simulink model "Quadrotor_Model"  (R2024b)
settings: Solver=ode45  StartTime=0.0  StopTime=350  RelTol=1e-3  EnableMultiTasking=on
values from neighbouring files (symbols this model uses):
  b = 0.07    [project_launch.m]
  g = 9.81    [project_launch.m]
  Ixx = 0.03411283500000001    (= 0.034112835)    [project_launch.m]
  Iyy = Ixx    (= 0.034112835)    [project_launch.m]
  Izz = 0.06314503500000002    (= 0.063145035)    [project_launch.m]
  Jr = 1.6129e-05    [project_launch.m]
  k = 0.09    [project_launch.m]
  K_d_phi = 0.01    [project_launch.m]
  K_d_psi = 0.136    [project_launch.m]
  K_d_theta = 0.1    [project_launch.m]
  K_dx = 0.00001    (= 1e-05)    [project_launch.m]
  K_dy = 0.00005    (= 5e-05)    [project_launch.m]
  K_dz = 0.001    [project_launch.m]
  K_p_phi = 0.05    [project_launch.m]
  K_p_psi = 0.4    [project_launch.m]
  K_p_theta = 0.0002    [project_launch.m]
  K_px = 0.00003    (= 3e-05)    [project_launch.m]
  K_py = 0.0001    [project_launch.m]
  K_pz = 0.0001    [project_launch.m]
  L = 0.381    [project_launch.m]
  m = 1.8    [project_launch.m]
settings Model: Creator=boyan  LastModifiedBy=Akhil Jarodia
settings SolverCC: MaxConsecutiveMinStep=2  AlgebraicLoopSolver=TrustRegion
settings DataIOCC: LimitDataPoints=on  SaveFormat=Array  ReturnWorkspaceOutputs=off
settings OptimizationCC: LifeSpan=inf
settings DebuggingCC: SolverPrmCheckMsg=warning  UnconnectedInputMsg=warning  UnconnectedOutputMsg=warning  UnconnectedLineMsg=warning  SFUnexpectedBacktrackingDiag=warning  SFNoUnconditionalDefaultTransitionDiag=warning  SFExecutionAtInitializationDiag=none  ArithmeticOperatorsInVariantConditions=warning
settings HardwareCC: ProdBitPerPointer=32  ProdBitPerSizeT=32  ProdBitPerPtrDiffT=32  ProdLargestAtomicFloat=None  ProdIntDivRoundTo=Undefined  ProdEndianess=Unspecified  ProdWordSize=32  ProdHWDeviceType=32-bit Generic
settings ModelReferenceCC: EnableRefExpFcnMdlSchedulingChecks=on  PropagateSignalLabelsOutOfModel=off
settings SFSimCC: SimUseLocalCustomCode=off  CustomCodeUndefinedFunction=UseInterfaceOnly
settings RTWCC: RTWUseLocalCustomCode=off  GPUComputeCapability=3.5  DLArmComputeVersion=19.05
settings CodeAppCC: StateflowObjectComments=on
settings GRTTargetCC: TargetLangStandard=C89/C90 (ANSI)
settings ConfigComp: CovMetricSettings=dw  CovSaveCumulativeToWorkspaceVar=on  CovSaveSingleToWorkspaceVar=on  CovExternalEMLEnable=off  CovSFcnEnable=off

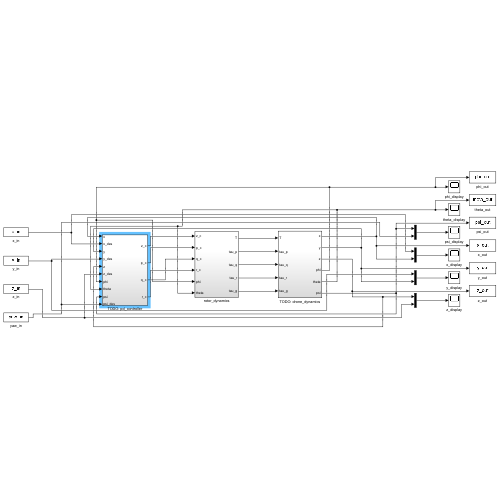
[thumbnail: Simulink's stored preview of the top-level diagram]
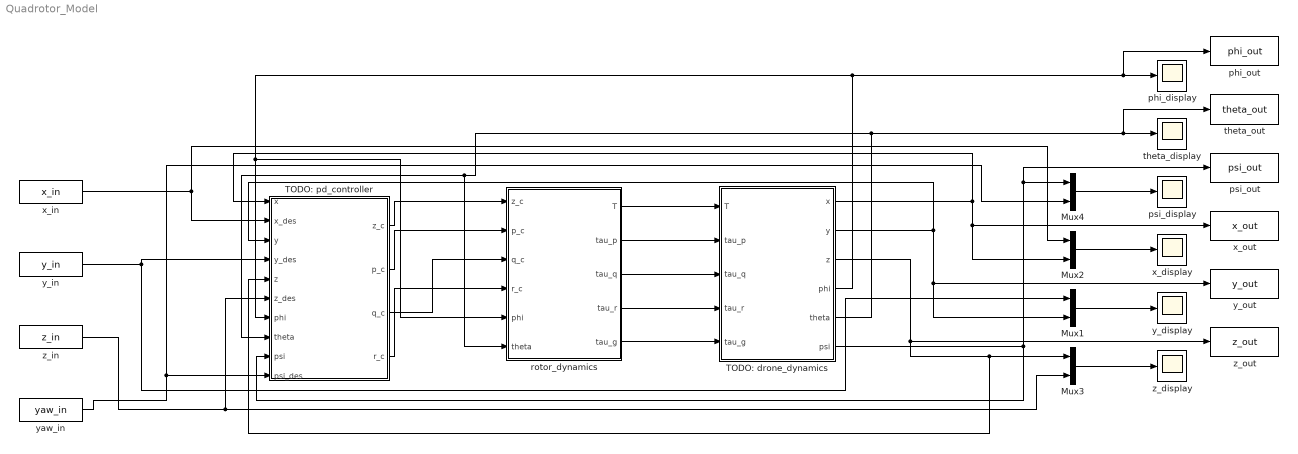
== system Quadrotor_Model ==
  Mux{1..4} (4 alike) : Mux  Inputs=2
  TODO: drone_dynamics : Subsystem
  TODO: pd_controller : Subsystem
  phi_display : Scope
  phi_out : ToWorkspace  VariableName=phi_out  SaveFormat=Timeseries  SampleTime=-1
  psi_display : Scope
  psi_out : ToWorkspace  VariableName=psi_out  SaveFormat=Timeseries  SampleTime=-1
  rotor_dynamics : Subsystem
  theta_display : Scope
  theta_out : ToWorkspace  VariableName=theta_out  SaveFormat=Timeseries  SampleTime=-1
  x_display : Scope
  x_in : FromWorkspace  VariableName=x_in
  x_out : ToWorkspace  VariableName=x_out  SaveFormat=Timeseries  SampleTime=-1
  y_display : Scope
  y_in : FromWorkspace  VariableName=y_in
  y_out : ToWorkspace  VariableName=y_out  SaveFormat=Timeseries  SampleTime=-1
  yaw_in : FromWorkspace  VariableName=yaw_in
  z_display : Scope
  z_in : FromWorkspace  VariableName=z_in
  z_out : ToWorkspace  VariableName=z_out  SaveFormat=Timeseries  SampleTime=-1
  wires:
  rotor_dynamics/1(T) -> TODO: drone_dynamics/1(T)
  rotor_dynamics/2(tau_p) -> TODO: drone_dynamics/2(tau_p)
  TODO: pd_controller/1(z_c) -> rotor_dynamics/1(z_c)
  TODO: pd_controller/2(p_c) -> rotor_dynamics/2(p_c)
  z_in/1 -> TODO: pd_controller/6(z_des), Mux3/2
  Mux1/1 -> y_display/1
  Mux2/1 -> x_display/1
  Mux4/1 -> psi_display/1
  Mux3/1 -> z_display/1
  TODO: drone_dynamics/6(psi) -> TODO: pd_controller/9(psi), psi_out/1, Mux4/1
  y_in/1 -> TODO: pd_controller/4(y_des), Mux1/1
  x_in/1 -> TODO: pd_controller/2(x_des), Mux2/1
  TODO: drone_dynamics/3(z) -> z_out/1, TODO: pd_controller/5(z), Mux3/1
  TODO: drone_dynamics/5(theta) -> theta_out/1, theta_display/1, rotor_dynamics/6(theta), TODO: pd_controller/8(theta)
  TODO: drone_dynamics/2(y) -> TODO: pd_controller/3(y), Mux1/2, y_out/1
  TODO: drone_dynamics/4(phi) -> phi_out/1, phi_display/1, rotor_dynamics/5(phi), TODO: pd_controller/7(phi)
  TODO: drone_dynamics/1(x) -> TODO: pd_controller/1(x), Mux2/2, x_out/1
  rotor_dynamics/5(tau_g) -> TODO: drone_dynamics/5(tau_g)
  rotor_dynamics/3(tau_q) -> TODO: drone_dynamics/3(tau_q)
  rotor_dynamics/4(tau_r) -> TODO: drone_dynamics/4(tau_r)
  yaw_in/1 -> Mux4/2, TODO: pd_controller/10(psi_des)
  TODO: pd_controller/4(r_c) -> rotor_dynamics/4(r_c)
  TODO: pd_controller/3(q_c) -> rotor_dynamics/3(q_c)

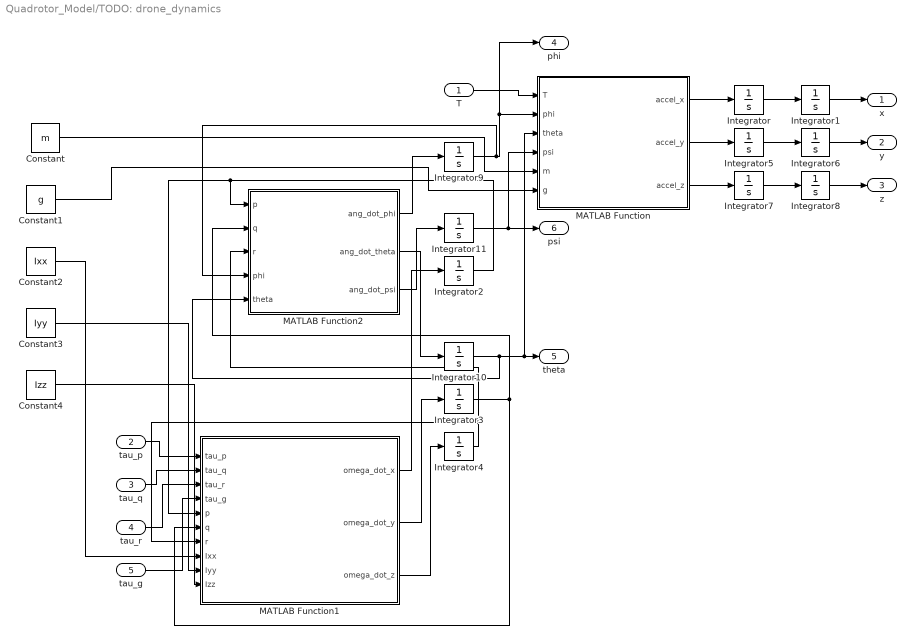
== system Quadrotor_Model/TODO: drone_dynamics ==
  T : Inport
  tau_p : Inport  Port=2
  tau_q : Inport  Port=3
  tau_r : Inport  Port=4
  tau_g : Inport  Port=5
  Constant : Constant  Value=m
  Constant1 : Constant  Value=g
  Constant2 : Constant  Value=Ixx
  Constant3 : Constant  Value=Iyy
  Constant4 : Constant  Value=Izz
  Integrator{,1..11} (12 alike) : Integrator
  MATLAB Function : MATLAB Function  TreatAsAtomicUnit=on
  MATLAB Function1 : MATLAB Function  TreatAsAtomicUnit=on
  MATLAB Function2 : MATLAB Function  TreatAsAtomicUnit=on
  x : Outport
  y : Outport  Port=2
  z : Outport  Port=3
  phi : Outport  Port=4
  theta : Outport  Port=5
  psi : Outport  Port=6
  wires:
  tau_p/1 -> MATLAB Function1/1(tau_p)
  tau_q/1 -> MATLAB Function1/2(tau_q)
  tau_r/1 -> MATLAB Function1/3(tau_r)
  tau_g/1 -> MATLAB Function1/4(tau_g)
  MATLAB Function2/3(ang_dot_psi) -> Integrator11/1
  MATLAB Function2/2(ang_dot_theta) -> Integrator10/1
  T/1 -> MATLAB Function/1(T)
  MATLAB Function2/1(ang_dot_phi) -> Integrator9/1
  MATLAB Function1/1(omega_dot_x) -> Integrator2/1
  MATLAB Function1/2(omega_dot_y) -> Integrator3/1
  MATLAB Function1/3(omega_dot_z) -> Integrator4/1
  Integrator9/1 -> phi/1, MATLAB Function/2(phi), MATLAB Function2/4(phi)
  Integrator5/1 -> Integrator6/1
  Integrator11/1 -> psi/1, MATLAB Function/4(psi)
  Integrator2/1 -> MATLAB Function1/5(p), MATLAB Function2/1(p)
  Integrator10/1 -> theta/1, MATLAB Function/3(theta), MATLAB Function2/5(theta)
  Integrator3/1 -> MATLAB Function2/2(q), MATLAB Function1/6(q)
  Integrator4/1 -> MATLAB Function1/7(r), MATLAB Function2/3(r)
  MATLAB Function/1(accel_x) -> Integrator/1
  MATLAB Function/2(accel_y) -> Integrator5/1
  MATLAB Function/3(accel_z) -> Integrator7/1
  Integrator/1 -> Integrator1/1
  Integrator7/1 -> Integrator8/1
  Integrator1/1 -> x/1
  Integrator6/1 -> y/1
  Integrator8/1 -> z/1
  Constant/1 -> MATLAB Function/5(m)
  Constant1/1 -> MATLAB Function/6(g)
  Constant2/1 -> MATLAB Function1/8(Ixx)
  Constant3/1 -> MATLAB Function1/9(Iyy)
  Constant4/1 -> MATLAB Function1/10(Izz)

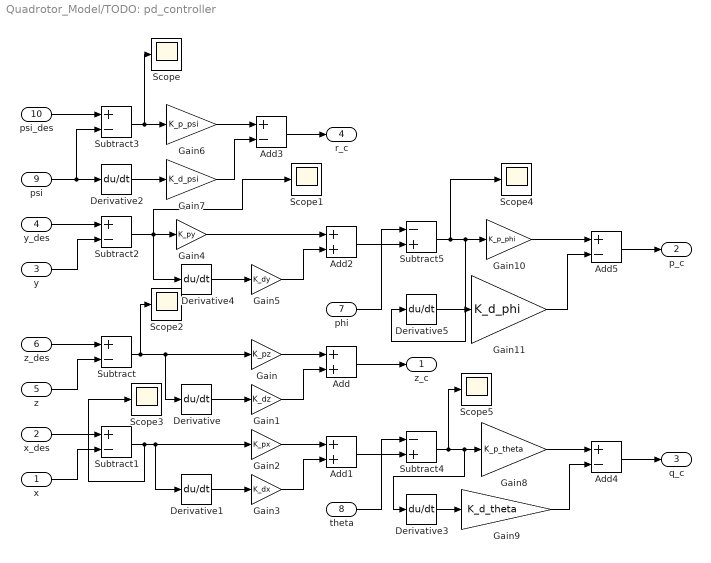
== system Quadrotor_Model/TODO: pd_controller ==
  x : Inport
  x_des : Inport  Port=2
  y : Inport  Port=3
  y_des : Inport  Port=4
  z : Inport  Port=5
  z_des : Inport  Port=6
  phi : Inport  Port=7
  theta : Inport  Port=8
  psi : Inport  Port=9
  psi_des : Inport  Port=10
  Add : Sum
  Add1 : Sum
  Add2 : Sum
  Add3 : Sum  Inputs=+-
  Add4 : Sum  Inputs=+-
  Add5 : Sum  Inputs=+-
  Derivative{,1..5} (6 alike) : Derivative
  Gain : Gain  Gain=K_pz
  Gain1 : Gain  Gain=K_dz
  Gain10 : Gain  Gain=K_p_phi
  Gain11 : Gain  Gain=K_d_phi
  Gain2 : Gain  Gain=K_px
  Gain3 : Gain  Gain=K_dx
  Gain4 : Gain  Gain=K_py
  Gain5 : Gain  Gain=K_dy
  Gain6 : Gain  Gain=K_p_psi
  Gain7 : Gain  Gain=K_d_psi
  Gain8 : Gain  Gain=K_p_theta
  Gain9 : Gain  Gain=K_d_theta
  Scope{,1..5} (6 alike) : Scope
  Subtract{,1..3} (4 alike) : Sum  Inputs=+-
  Subtract4 : Sum  Inputs=-+
  Subtract5 : Sum  Inputs=-+
  z_c : Outport
  p_c : Outport  Port=2
  q_c : Outport  Port=3
  r_c : Outport  Port=4
  wires:
  Add2/1 -> Subtract5/2
  psi/1 -> Subtract3/2, Derivative2/1
  x/1 -> Subtract1/2
  psi_des/1 -> Subtract3/1
  z_des/1 -> Subtract/1
  phi/1 -> Subtract5/1
  y/1 -> Subtract2/2
  y_des/1 -> Subtract2/1
  x_des/1 -> Subtract1/1
  z/1 -> Subtract/2
  Add1/1 -> Subtract4/2
  Subtract1/1 -> Scope3/1, Gain2/1, Derivative1/1
  Subtract3/1 -> Scope/1, Gain6/1
  Add/1 -> z_c/1
  Derivative2/1 -> Gain7/1
  Gain10/1 -> Add5/1
  Subtract/1 -> Scope2/1, Gain/1, Derivative/1
  Subtract2/1 -> Scope1/1, Gain4/1, Derivative4/1
  Gain6/1 -> Add3/1
  Gain7/1 -> Add3/2
  Gain4/1 -> Add2/1
  Derivative4/1 -> Gain5/1
  Derivative/1 -> Gain1/1
  Derivative1/1 -> Gain3/1
  Add3/1 -> r_c/1
  Gain5/1 -> Add2/2
  Gain/1 -> Add/1
  Gain3/1 -> Add1/2
  Gain1/1 -> Add/2
  Gain2/1 -> Add1/1
  theta/1 -> Subtract4/1
  Gain9/1 -> Add4/2
  Subtract5/1 -> Scope4/1, Derivative5/1, Gain10/1
  Derivative5/1 -> Gain11/1
  Gain11/1 -> Add5/2
  Subtract4/1 -> Scope5/1, Derivative3/1, Gain8/1
  Derivative3/1 -> Gain9/1
  Gain8/1 -> Add4/1
  Add5/1 -> p_c/1
  Add4/1 -> q_c/1

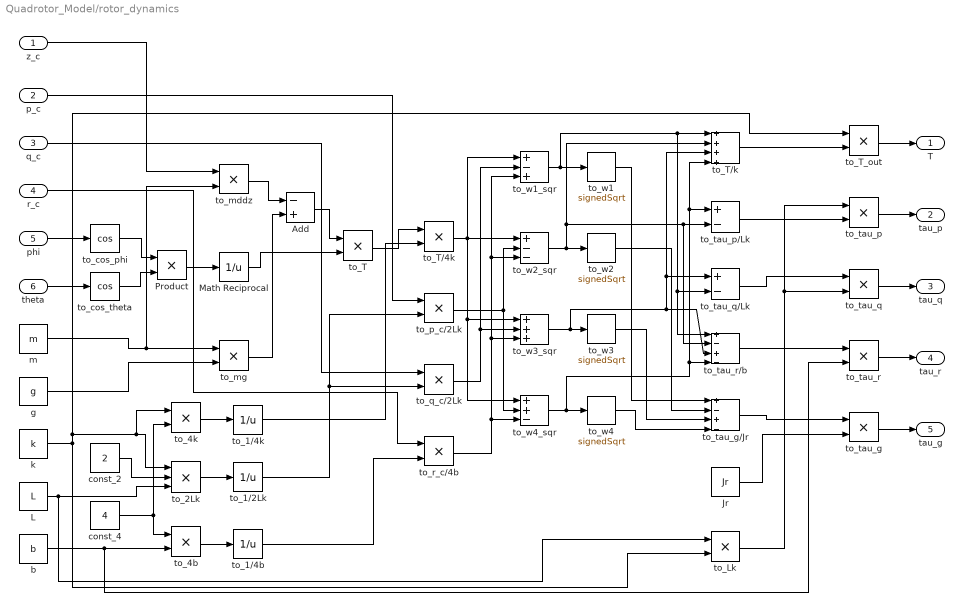
== system Quadrotor_Model/rotor_dynamics ==
  z_c : Inport
  p_c : Inport  Port=2
  q_c : Inport  Port=3
  r_c : Inport  Port=4
  phi : Inport  Port=5
  theta : Inport  Port=6
  Add : Sum  Inputs=-+
  Jr : Constant  Value=Jr
  L : Constant  Value=L
  Math Reciprocal : Math  Operator=reciprocal  SignedPower=on
  Product : Product
  b : Constant  Value=b
  const_2 : Constant  Value=2
  const_4 : Constant  Value=4
  g : Constant  Value=g
  k : Constant  Value=k
  m : Constant  Value=m
  to_1/2Lk : Math  Operator=reciprocal  SignedPower=on
  to_1/4b : Math  Operator=reciprocal  SignedPower=on
  to_1/4k : Math  Operator=reciprocal  SignedPower=on
  to_2Lk : Product  Inputs=3
  to_4b : Product
  to_4k : Product
  to_Lk : Product
  to_T : Product
  to_T/4k : Product
  to_T/k : Sum  Inputs=++++
  to_T_out : Product
  to_cos_phi : Trigonometry  Operator=cos
  to_cos_theta : Trigonometry  Operator=cos
  to_mddz : Product
  to_mg : Product
  to_p_c/2Lk : Product
  to_q_c/2Lk : Product
  to_r_c/4b : Product
  to_tau_g : Product
  to_tau_g/Jr : Sum  Inputs=+-+-
  to_tau_p : Product
  to_tau_p/Lk : Sum  Inputs=+-
  to_tau_q : Product
  to_tau_q/Lk : Sum  Inputs=+-
  to_tau_r : Product
  to_tau_r/b : Sum  Inputs=+-+-
  to_w{1..4} (4 alike) : Sqrt  Operator=signedSqrt
  to_w1_sqr : Sum  Inputs=+-+
  to_w2_sqr : Sum  Inputs=+--
  to_w3_sqr : Sum  Inputs=+++
  to_w4_sqr : Sum  Inputs=++-
  T : Outport
  tau_p : Outport  Port=2
  tau_q : Outport  Port=3
  tau_r : Outport  Port=4
  tau_g : Outport  Port=5
  wires:
  phi/1 -> to_cos_phi/1
  theta/1 -> to_cos_theta/1
  to_cos_phi/1 -> Product/1
  to_cos_theta/1 -> Product/2
  Product/1 -> Math Reciprocal/1
  m/1 -> to_mddz/2, to_mg/1
  g/1 -> to_mg/2
  to_mg/1 -> Add/2
  Math Reciprocal/1 -> to_T/2
  Add/1 -> to_T/1
  k/1 -> to_2Lk/1, to_4k/1, to_T_out/1, to_Lk/2
  const_4/1 -> to_4b/1, to_4k/2
  const_2/1 -> to_2Lk/2
  L/1 -> to_2Lk/3, to_Lk/1
  b/1 -> to_tau_r/2, to_4b/2
  to_4k/1 -> to_1/4k/1
  to_2Lk/1 -> to_1/2Lk/1
  to_4b/1 -> to_1/4b/1
  to_T/1 -> to_T/4k/1
  to_1/4k/1 -> to_T/4k/2
  p_c/1 -> to_p_c/2Lk/1
  to_1/2Lk/1 -> to_q_c/2Lk/2, to_p_c/2Lk/2
  q_c/1 -> to_q_c/2Lk/1
  to_1/4b/1 -> to_r_c/4b/2
  r_c/1 -> to_r_c/4b/1
  to_T/4k/1 -> to_w2_sqr/1, to_w3_sqr/1, to_w4_sqr/1, to_w1_sqr/1
  to_q_c/2Lk/1 -> to_w3_sqr/2, to_w1_sqr/2
  to_r_c/4b/1 -> to_w4_sqr/3, to_w3_sqr/3, to_w2_sqr/3, to_w1_sqr/3
  to_p_c/2Lk/1 -> to_w2_sqr/2, to_w4_sqr/2
  to_w1_sqr/1 -> to_w1/1, to_tau_r/b/1, to_tau_q/Lk/2, to_T/k/1
  to_w2_sqr/1 -> to_w2/1, to_tau_r/b/2, to_tau_p/Lk/2, to_T/k/2
  to_w3_sqr/1 -> to_w3/1, to_tau_q/Lk/1, to_T/k/3, to_tau_r/b/3
  to_w4_sqr/1 -> to_w4/1, to_tau_p/Lk/1, to_T/k/4, to_tau_r/b/4
  to_w2/1 -> to_tau_g/Jr/2
  to_w1/1 -> to_tau_g/Jr/1
  to_w3/1 -> to_tau_g/Jr/3
  to_w4/1 -> to_tau_g/Jr/4
  to_T_out/1 -> T/1
  to_T/k/1 -> to_T_out/2
  to_tau_p/1 -> tau_p/1
  to_tau_p/Lk/1 -> to_tau_p/2
  to_tau_q/1 -> tau_q/1
  to_tau_r/1 -> tau_r/1
  to_tau_r/b/1 -> to_tau_r/1
  to_tau_q/Lk/1 -> to_tau_q/1
  to_tau_g/1 -> tau_g/1
  to_tau_g/Jr/1 -> to_tau_g/1
  to_Lk/1 -> to_tau_p/1, to_tau_q/2
  Jr/1 -> to_tau_g/2
  z_c/1 -> to_mddz/1
  to_mddz/1 -> Add/1

== matlab function Quadrotor_Model/TODO: drone_dynamics/MATLAB Function1 ==
  data: tau_p input; omega_dot_x output; tau_q input; tau_r input; tau_g input; p input; q input; r input; omega_dot_y output; omega_dot_z output; Ixx input; Iyy input; Izz input
function [omega_dot_x, omega_dot_y, omega_dot_z] = rotational_dynamics(tau_p, tau_q, tau_r, tau_g, p, q, r, Ixx, Iyy, Izz)
    % Rotational Dynamics
    % Inputs:
    %   tau_p, tau_q, tau_r - Torques about x, y, z axes (Nm)
    %   tau_g               - Gyroscopic torque (Nm)
    %   p, q, r             - Angular velocities about x, y, z axes (rad/s)
    %   Ixx, Iyy, Izz       - Moments of inertia (kg·m^2)
    % Outputs:
    %   omega_dot           - Angular accelerations [dp/dt, dq/dt, dr/dt] (rad/s^2)

    % Compute angular accelerations
    omega_dot_x = (1 / Ixx) * (tau_p - tau_g * q + (Iyy - Izz) * q * r);
    omega_dot_y = (1 / Iyy) * (tau_q - tau_g * p + (Izz - Ixx) * p * r);
    omega_dot_z = (1 / Izz) * (tau_r + (Ixx - Iyy) * p * q);
end

== matlab function Quadrotor_Model/TODO: drone_dynamics/MATLAB Function ==
  data: T input; phi input; theta input; psi input; accel_x output; accel_y output; accel_z output; m input; g input
function [accel_x, accel_y, accel_z] = translational_dynamics(T, phi, theta, psi, m, g)
    % Translational Dynamics
    % Inputs:
    %   T     - Thrust (N)
    %   phi   - Roll angle (rad)
    %   theta - Pitch angle (rad)
    %   psi   - Yaw angle (rad)
    %   m     - Mass of the drone (kg)
    %   g     - Gravitational acceleration (m/s^2)
    % Outputs:
    %   accel - Translational accelerations [ddot_x, ddot_y, ddot_z] (m/s^2)
    % Compute translational accelerations
    accel_x = (T / m) * (cos(psi) * sin(theta) * cos(phi) + sin(psi) * sin(phi));
    accel_y = (T / m) * (sin(psi) * sin(theta) * cos(phi) - cos(psi) * sin(phi));
    accel_z = (T / m) * (cos(theta) * cos(phi)) - g;
end

== matlab function Quadrotor_Model/TODO: drone_dynamics/MATLAB Function2 ==
  data: p input; ang_dot_phi output; q input; r input; phi input; theta input; ang_dot_theta output; ang_dot_psi output
function [ang_dot_phi, ang_dot_theta, ang_dot_psi] = euler_angle_dynamics(p, q, r, phi, theta)
    % Euler Angle Dynamics
    % Inputs:
    %   p, q, r   - Angular velocities about x, y, z axes (rad/s)
    %   phi, theta - Roll and pitch angles (rad)
    % Outputs:
    %   ang_dot   - Euler angle rates [dphi/dt, dtheta/dt, dpsi/dt] (rad/s)

    % Compute Euler angle derivatives
    ang_dot_phi = p + q * sin(phi) * tan(theta) + r * cos(phi) * tan(theta);
    ang_dot_theta = q * cos(phi) - r * sin(phi);
    ang_dot_psi = q * sin(phi) / cos(theta) + r * cos(phi) / cos(theta);
end
